simulink model "SystemModeDeterminationComponent"  (R2026a)
settings: Solver=FixedStepDiscrete
settings Model: DataDictionary=TractionEmotorSoftwareArchInterfaceData.sldd  Creator=dakaihu  LastModifiedBy=dakaihu

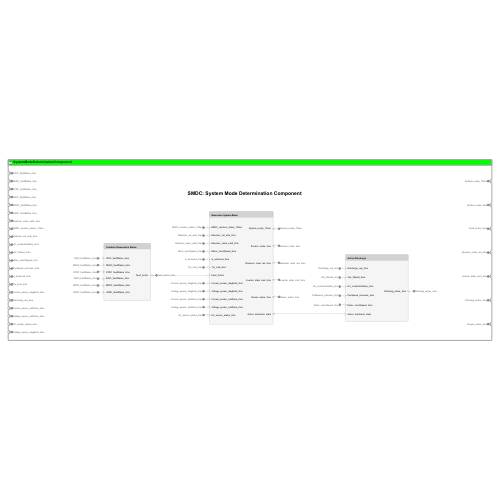
[thumbnail: Simulink's stored preview of the top-level diagram]
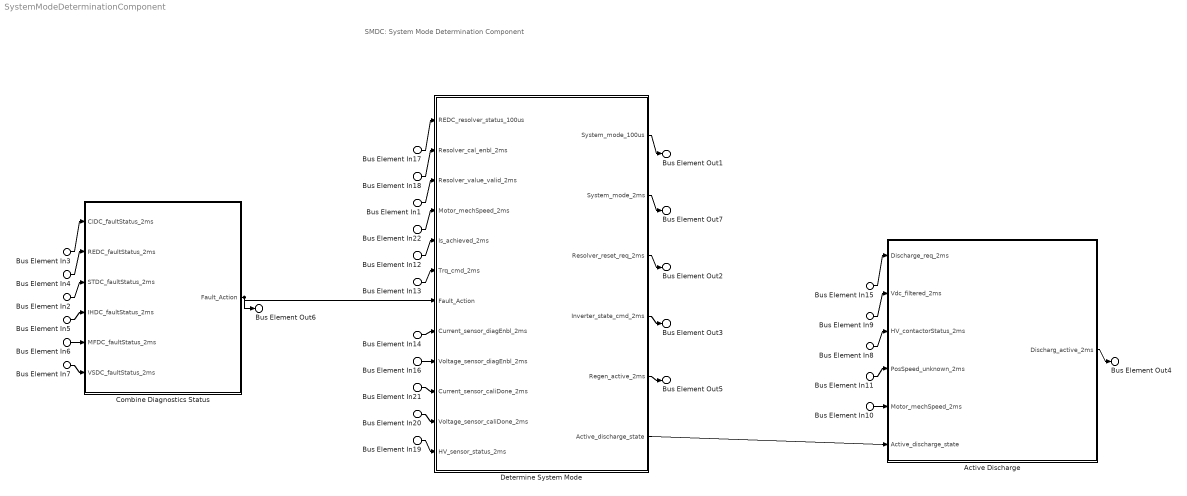
== system SystemModeDeterminationComponent ==
  note: SMDC: System Mode Determination Component
  Bus Element In3 : Inport  PortName=CIDC_faultStatus_2ms
  Bus Element In4 : Inport  Port=2  PortName=REDC_faultStatus_2ms
  Bus Element In2 : Inport  Port=3  PortName=STDC_faultStatus_2ms
  Bus Element In5 : Inport  Port=4  PortName=IHDC_faultStatus_2ms
  Bus Element In6 : Inport  Port=5  PortName=MFDC_faultStatus_2ms
  Bus Element In7 : Inport  Port=6  PortName=VSDC_faultStatus_2ms
  Bus Element In1 : Inport  Port=7  PortName=Resolver_value_valid_2ms
  Bus Element In17 : Inport  Port=8  PortName=REDC_resolver_status_100us
  Bus Element In18 : Inport  Port=9  PortName=Resolver_cal_enbl_2ms
  Bus Element In8 : Inport  Port=10  PortName=HV_contactorStatus_2ms
  Bus Element In9 : Inport  Port=11  PortName=Vdc_filtered_2ms
  Bus Element In10 : Inport  Port=12  PortName=Motor_mechSpeed_2ms
  Bus Element In22 : Inport  Port=12  PortName=Motor_mechSpeed_2ms
  Bus Element In11 : Inport  Port=13  PortName=PosSpeed_unknown_2ms
  Bus Element In12 : Inport  Port=14  PortName=Is_achieved_2ms
  Bus Element In13 : Inport  Port=15  PortName=Trq_cmd_2ms
  Bus Element In14 : Inport  Port=16  PortName=Current_sensor_diagEnbl_2ms
  Bus Element In15 : Inport  Port=17  PortName=Discharge_req_2ms
  Bus Element In21 : Inport  Port=18  PortName=Current_sensor_caliDone_2ms
  Bus Element In20 : Inport  Port=19  PortName=Voltage_sensor_caliDone_2ms
  Bus Element In19 : Inport  Port=20  PortName=HV_sensor_status_2ms
  Bus Element In16 : Inport  Port=21  PortName=Voltage_sensor_diagEnbl_2ms
  Active Discharge : Subsystem
      settings: PortSchema="{\"entries\":[{\"content\":{\"headerSize\":26,\"margin\":15,\"minimumSpacing\":25,\"sides\":[{\"content\":{\"connectorIds\":[\"In1\",\"In2\",\"In3\",\"In4\",\"In5\",\"In6\"]},\"type\":\"ConnectorPlacement.EquallySpacedRectSide\",\"uuid\":\"b2f30fca-3d8e-46ee-af1d-282b22b9b844\"},{\"content\":{\"connectorIds\":[\"Out1\"],\"side\":\"RIGHT\"},\"type\":\"ConnectorPlacement.EquallySpacedRectSide\",\"uuid\":\"2d7d706d-eac4-4c73-84e8-2a36a393a616\"},{\"content\":{\"connectorIds\":[],\"side\":\"TOP\"},\"type\":\"ConnectorPlacement.EquallySpacedRectSide\",\"uuid\":\"b52ae510-b7cc-4ed0-8d34-4a095deae41b\"}]},\"type\":\"ConnectorPlacement.EquallySpacedConnector\",\"uuid\":\"1257e7cc-1858-4bc4-ab05-7b00060cf0d5\"}],\"packageUris\":[\"http://schema.mathworks.com/mf0/Connector/R2020b\"],\"version\":\"1.0\"}"
  Combine Diagnostics Status : Subsystem
      settings: PortSchema="{\"entries\":[{\"content\":{\"headerSize\":26,\"margin\":15,\"minimumSpacing\":25,\"sides\":[{\"content\":{\"connectorIds\":[\"In1\",\"In2\",\"In3\",\"In4\",\"In5\",\"In6\"]},\"type\":\"ConnectorPlacement.EquallySpacedRectSide\",\"uuid\":\"b2f30fca-3d8e-46ee-af1d-282b22b9b844\"},{\"content\":{\"connectorIds\":[\"Out1\"],\"side\":\"RIGHT\"},\"type\":\"ConnectorPlacement.EquallySpacedRectSide\",\"uuid\":\"2d7d706d-eac4-4c73-84e8-2a36a393a616\"},{\"content\":{\"connectorIds\":[],\"side\":\"TOP\"},\"type\":\"ConnectorPlacement.EquallySpacedRectSide\",\"uuid\":\"b52ae510-b7cc-4ed0-8d34-4a095deae41b\"}]},\"type\":\"ConnectorPlacement.EquallySpacedConnector\",\"uuid\":\"1257e7cc-1858-4bc4-ab05-7b00060cf0d5\"}],\"packageUris\":[\"http://schema.mathworks.com/mf0/Connector/R2020b\"],\"version\":\"1.0\"}"
  Determine System Mode : Subsystem
      settings: PortSchema="{\"entries\":[{\"content\":{\"headerSize\":26,\"margin\":15,\"minimumSpacing\":25,\"sides\":[{\"content\":{\"connectorIds\":[\"In4\",\"In3\",\"In2\",\"In5\",\"In6\",\"In7\",\"In1\",\"In8\",\"In9\",\"In10\",\"In11\",\"In12\"]},\"type\":\"ConnectorPlacement.EquallySpacedRectSide\",\"uuid\":\"b2f30fca-3d8e-46ee-af1d-282b22b9b844\"},{\"content\":{\"connectorIds\":[\"Out1\",\"Out2\",\"Out3\",\"Out4\",\"Out5\",\"Out6\"],\"side\":\"RIGHT\"},\"type\":\"ConnectorPlacement.EquallySpacedRectSide\",\"uuid\":\"2d7d706d-eac4-4c73-84e8-2a36a393a616\"},{\"content\":{\"connectorIds\":[],\"side\":\"TOP\"},\"type\":\"ConnectorPlacement.EquallySpacedRectSide\",\"uuid\":\"b52ae510-b7cc-4ed0-8d34-4a095deae41b\"}]},\"type\":\"ConnectorPlacement.EquallySpacedConnector\",\"uuid\":\"1257e7cc-1858-4bc4-ab05-7b00060cf0d5\"}],\"packageUris\":[\"http://schema.mathworks.com/mf0/Connector/R2020b\"],\"version\":\"1.0\"}"
  Bus Element Out1 : Outport  PortName=System_mode_100us
  Bus Element Out7 : Outport  Port=2  PortName=System_mode_2ms
  Bus Element Out6 : Outport  Port=3  PortName=Fault_action_2ms
  Bus Element Out2 : Outport  Port=4  PortName=Resolver_reset_req_2ms
  Bus Element Out3 : Outport  Port=5  PortName=Inverter_state_cmd_2ms
  Bus Element Out4 : Outport  Port=6  PortName=Discharg_active_2ms
  Bus Element Out5 : Outport  Port=7  PortName=Regen_active_2ms
  wires:
  Bus Element In3/1 -> Combine Diagnostics Status/1(CIDC_faultStatus_2ms)
  Bus Element In4/1 -> Combine Diagnostics Status/2(REDC_faultStatus_2ms)
  Bus Element In2/1 -> Combine Diagnostics Status/3(STDC_faultStatus_2ms)
  Bus Element In5/1 -> Combine Diagnostics Status/4(IHDC_faultStatus_2ms)
  Bus Element In6/1 -> Combine Diagnostics Status/5(MFDC_faultStatus_2ms)
  Bus Element In7/1 -> Combine Diagnostics Status/6(VSDC_faultStatus_2ms)
  Combine Diagnostics Status/1(Fault_Action) -> Determine System Mode/1(Fault_Action), Bus Element Out6/1
  Bus Element In15/1 -> Active Discharge/1(Discharge_req_2ms)
  Bus Element In9/1 -> Active Discharge/2(Vdc_filtered_2ms)
  Bus Element In8/1 -> Active Discharge/3(HV_contactorStatus_2ms)
  Bus Element In11/1 -> Active Discharge/4(PosSpeed_unknown_2ms)
  Bus Element In1/1 -> Determine System Mode/2(Resolver_value_valid_2ms)
  Bus Element In17/1 -> Determine System Mode/4(REDC_resolver_status_100us)
  Bus Element In18/1 -> Determine System Mode/3(Resolver_cal_enbl_2ms)
  Bus Element In10/1 -> Active Discharge/5(Motor_mechSpeed_2ms)
  Bus Element In22/1 -> Determine System Mode/5(Motor_mechSpeed_2ms)
  Bus Element In12/1 -> Determine System Mode/6(Is_achieved_2ms)
  Bus Element In13/1 -> Determine System Mode/7(Trq_cmd_2ms)
  Bus Element In14/1 -> Determine System Mode/8(Current_sensor_diagEnbl_2ms)
  Bus Element In16/1 -> Determine System Mode/9(Voltage_sensor_diagEnbl_2ms)
  Bus Element In21/1 -> Determine System Mode/10(Current_sensor_caliDone_2ms)
  Bus Element In20/1 -> Determine System Mode/11(Voltage_sensor_caliDone_2ms)
  Bus Element In19/1 -> Determine System Mode/12(HV_sensor_status_2ms)
  Determine System Mode/1(System_mode_100us) -> Bus Element Out1/1
  Determine System Mode/2(System_mode_2ms) -> Bus Element Out7/1
  Determine System Mode/3(Resolver_reset_req_2ms) -> Bus Element Out2/1
  Determine System Mode/4(Inverter_state_cmd_2ms) -> Bus Element Out3/1
  Active Discharge/1(Discharg_active_2ms) -> Bus Element Out4/1
  Determine System Mode/5(Regen_active_2ms) -> Bus Element Out5/1
  Determine System Mode/6(Active_discharge_state) -> Active Discharge/6(Active_discharge_state)

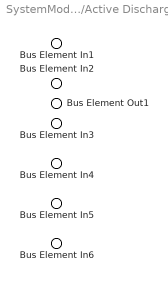
== system SystemModeDeterminationComponent/Active Discharge ==
  Bus Element In1 : Inport  PortName=Discharge_req_2ms
  Bus Element In2 : Inport  Port=2  PortName=Vdc_filtered_2ms
  Bus Element In3 : Inport  Port=3  PortName=HV_contactorStatus_2ms
  Bus Element In4 : Inport  Port=4  PortName=PosSpeed_unknown_2ms
  Bus Element In5 : Inport  Port=5  PortName=Motor_mechSpeed_2ms
  Bus Element In6 : Inport  Port=6  PortName=Active_discharge_state
  Bus Element Out1 : Outport  PortName=Discharg_active_2ms

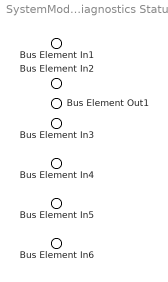
== system SystemModeDeterminationComponent/Combine Diagnostics Status ==
  Bus Element In1 : Inport  PortName=CIDC_faultStatus_2ms
  Bus Element In2 : Inport  Port=2  PortName=REDC_faultStatus_2ms
  Bus Element In3 : Inport  Port=3  PortName=STDC_faultStatus_2ms
  Bus Element In4 : Inport  Port=4  PortName=IHDC_faultStatus_2ms
  Bus Element In5 : Inport  Port=5  PortName=MFDC_faultStatus_2ms
  Bus Element In6 : Inport  Port=6  PortName=VSDC_faultStatus_2ms
  Bus Element Out1 : Outport  PortName=Fault_Action

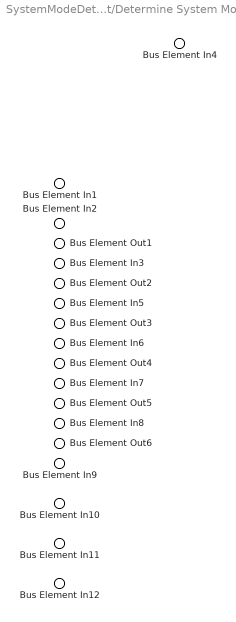
== system SystemModeDeterminationComponent/Determine System Mode ==
  Bus Element In1 : Inport  PortName=Fault_Action
  Bus Element In2 : Inport  Port=2  PortName=Resolver_value_valid_2ms
  Bus Element In4 : Inport  Port=3  PortName=Resolver_cal_enbl_2ms
  Bus Element In3 : Inport  Port=4  PortName=REDC_resolver_status_100us
  Bus Element In5 : Inport  Port=5  PortName=Motor_mechSpeed_2ms
  Bus Element In6 : Inport  Port=6  PortName=Is_achieved_2ms
  Bus Element In7 : Inport  Port=7  PortName=Trq_cmd_2ms
  Bus Element In8 : Inport  Port=8  PortName=Current_sensor_diagEnbl_2ms
  Bus Element In9 : Inport  Port=9  PortName=Voltage_sensor_diagEnbl_2ms
  Bus Element In10 : Inport  Port=10  PortName=Current_sensor_caliDone_2ms
  Bus Element In11 : Inport  Port=11  PortName=Voltage_sensor_caliDone_2ms
  Bus Element In12 : Inport  Port=12  PortName=HV_sensor_status_2ms
  Bus Element Out1 : Outport  PortName=System_mode_100us
  Bus Element Out2 : Outport  Port=2  PortName=System_mode_2ms
  Bus Element Out3 : Outport  Port=3  PortName=Resolver_reset_req_2ms
  Bus Element Out4 : Outport  Port=4  PortName=Inverter_state_cmd_2ms
  Bus Element Out5 : Outport  Port=5  PortName=Regen_active_2ms
  Bus Element Out6 : Outport  Port=6  PortName=Active_discharge_state
